simulink model "template"  (R2022b)
settings: Solver=VariableStepAuto  StartTime=0.0  StopTime=100  RelTol=1e-3
libraries: simulink_extras x3, aerolibanimutils x1, shared6dof x1
settings Model: Creator=alvar  LastModifiedBy=mluser

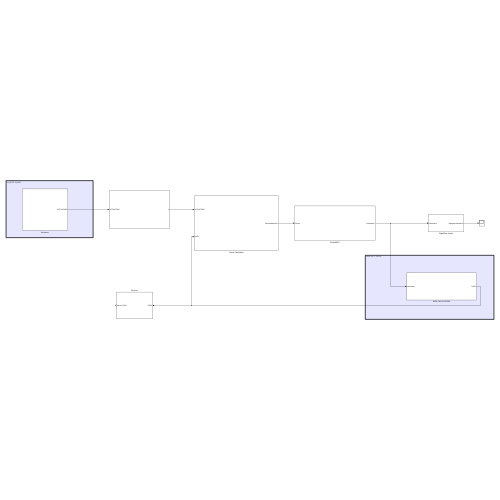
[thumbnail: Simulink's stored preview of the top-level diagram]
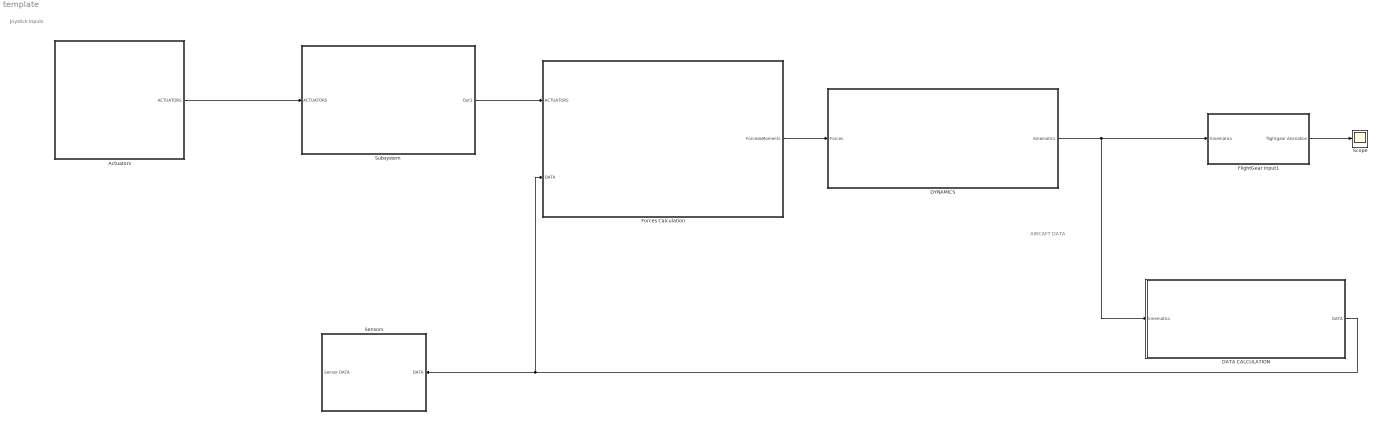
== system template ==
  note: Joystick Inputs
  note: AIRCAFT DATA
  Actuators : Subsystem
  DATA CALCULATION : Subsystem
  DYNAMICS : Subsystem
  FlightGear Input1 : Subsystem
  Forces Calculation : Subsystem
  Scope : Scope
  Sensors : Subsystem
  Subsystem : Subsystem
  wires:
  Forces Calculation/1(Forces&Moments) -> DYNAMICS/1(Forces)
  Actuators/1(ACTUATORS) -> Subsystem/1(ACTUATORS)
  DYNAMICS/1(Kinematics) -> FlightGear Input1/1(Kinematics), DATA CALCULATION/1(kinematics)
  DATA CALCULATION/1(DATA) -> Forces Calculation/2(DATA), Sensors/1(DATA)
  FlightGear Input1/1(flightgear Animation) -> Scope/1
  Subsystem/1(Out1) -> Forces Calculation/1(ACTUATORS)

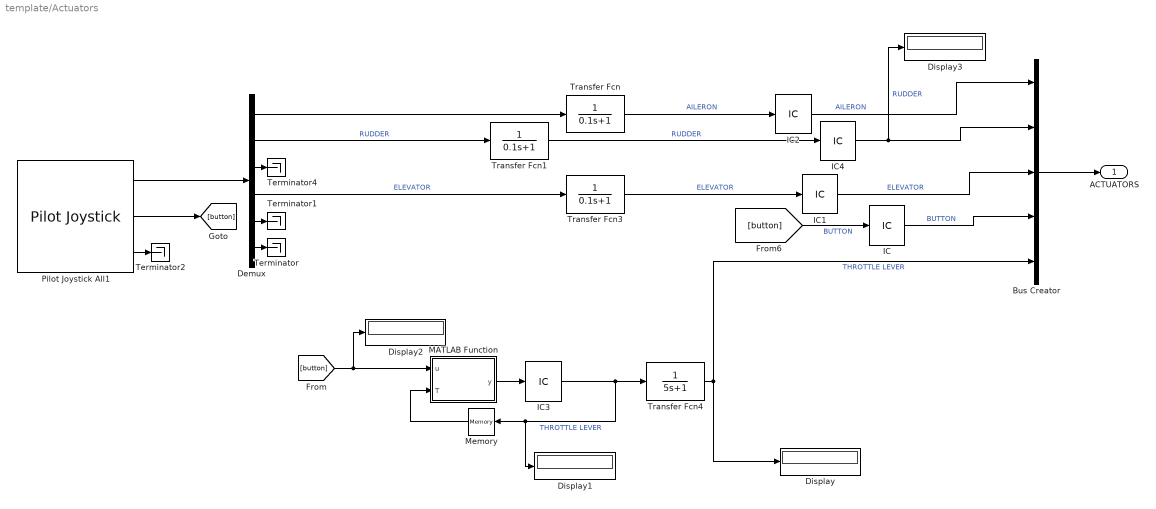
== system template/Actuators ==
  Bus Creator : BusCreator  Inputs=5
  Demux : Demux  Outputs=6
  Display{,1..3} (4 alike) : Display
  IC{,1..4} (5 alike) : InitialCondition  Value=0
  MATLAB Function : MATLAB Function  TreatAsAtomicUnit=on
  Memory : Memory
  Pilot Joystick All1 : aerolibanimutils/Pilot Joystick  JoystickID=Joystick1  OutputConfiguration=AllOutputs  SampleTime=1/30
      settings: LibrarySourceBlock=aerolibanimutils/Pilot Joystick All
  Terminator{,1..2,4} (4 alike) : Terminator
  Transfer Fcn : TransferFcn  Denominator=[0.1 1]
  Transfer Fcn1 : TransferFcn  Denominator=[0.1 1]
  Transfer Fcn3 : TransferFcn  Denominator=[0.1 1]
  Transfer Fcn4 : TransferFcn  Denominator=[5 1]
  ACTUATORS : Outport
  wires:
  Pilot Joystick All1/1 -> Demux/1
  Pilot Joystick All1/3 -> Terminator2/1
  Transfer Fcn3/1 -> IC1/1  "ELEVATOR"
  Pilot Joystick All1/2 -> [button]
  [button] -> IC/1  "BUTTON"
  Bus Creator/1 -> ACTUATORS/1
  IC/1 -> Bus Creator/4  "BUTTON"
  Transfer Fcn1/1 -> IC4/1  "RUDDER"
  Transfer Fcn/1 -> IC2/1  "AILERON"
  Demux/1 -> Transfer Fcn/1
  Demux/6 -> Terminator/1
  Demux/5 -> Terminator1/1
  Demux/4 -> Transfer Fcn3/1  "ELEVATOR"
  Demux/2 -> Transfer Fcn1/1  "RUDDER"
  Memory/1 -> MATLAB Function/2(T)
  IC3/1 -> Display1/1, Memory/1, Transfer Fcn4/1  "THROTTLE LEVER"
  MATLAB Function/1(y) -> IC3/1
  [button] -> Display2/1, MATLAB Function/1(u)
  Demux/3 -> Terminator4/1
  Transfer Fcn4/1 -> Display/1, Bus Creator/5  "THROTTLE LEVER"
  IC2/1 -> Bus Creator/1  "AILERON"
  IC4/1 -> Display3/1, Bus Creator/2  "RUDDER"
  IC1/1 -> Bus Creator/3  "ELEVATOR"

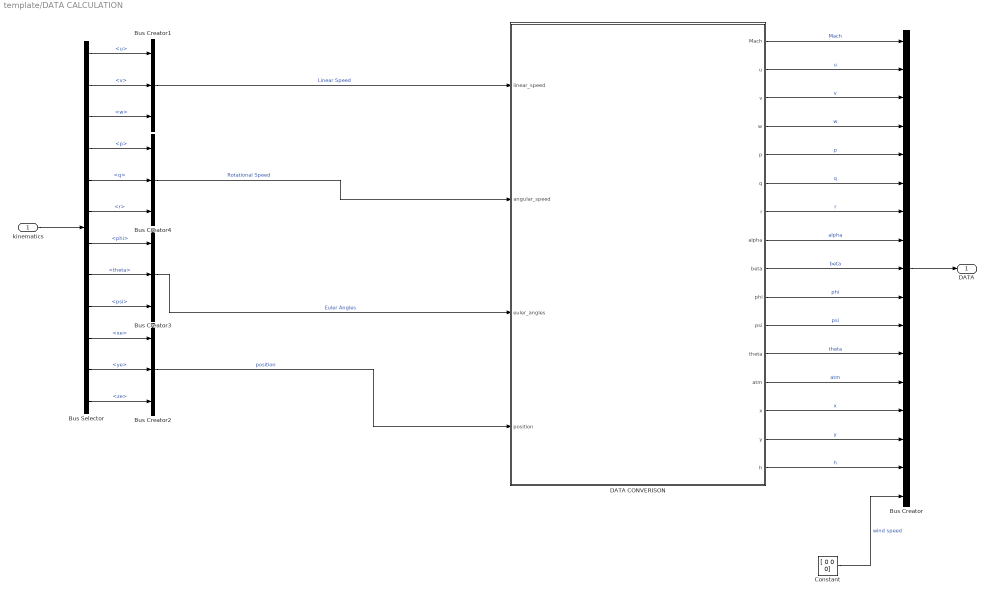
== system template/DATA CALCULATION ==
  kinematics : Inport
  Bus Creator : BusCreator  Inputs=17
  Bus Creator{1..4} (4 alike) : BusCreator  Inputs=3
  Bus Selector : BusSelector  OutputSignals=u,v,w,p,q,r,phi,theta,psi,xe,ye,ze
  Constant : Constant  Value=[ 0 0 0]
  DATA CONVERISON : MATLAB Function  TreatAsAtomicUnit=on
  DATA : Outport
  wires:
  kinematics/1 -> Bus Selector/1
  Bus Creator1/1 -> DATA CONVERISON/1(linear_speed)  "Linear Speed"
  Bus Creator4/1 -> DATA CONVERISON/2(angular_speed)  "Rotational Speed"
  Bus Creator3/1 -> DATA CONVERISON/3(euler_angles)  "Euler Angles"
  DATA CONVERISON/1(Mach) -> Bus Creator/1  "Mach"
  DATA CONVERISON/2(u) -> Bus Creator/2  "u"
  DATA CONVERISON/3(v) -> Bus Creator/3  "v"
  DATA CONVERISON/4(w) -> Bus Creator/4  "w"
  DATA CONVERISON/5(p) -> Bus Creator/5  "p"
  DATA CONVERISON/6(q) -> Bus Creator/6  "q"
  DATA CONVERISON/7(r) -> Bus Creator/7  "r"
  DATA CONVERISON/8(alpha) -> Bus Creator/8  "alpha"
  DATA CONVERISON/9(beta) -> Bus Creator/9  "beta"
  DATA CONVERISON/10(phi) -> Bus Creator/10  "phi"
  DATA CONVERISON/11(psi) -> Bus Creator/11  "psi"
  DATA CONVERISON/12(theta) -> Bus Creator/12  "theta"
  DATA CONVERISON/13(atm) -> Bus Creator/13  "atm"
  Bus Creator/1 -> DATA/1
  DATA CONVERISON/14(x) -> Bus Creator/14  "x"
  DATA CONVERISON/15(y) -> Bus Creator/15  "y"
  DATA CONVERISON/16(h) -> Bus Creator/16  "h"
  Bus Creator2/1 -> DATA CONVERISON/4(position)  "position"
  Bus Selector/1 -> Bus Creator1/1  "<u>"
  Bus Selector/2 -> Bus Creator1/2  "<v>"
  Bus Selector/3 -> Bus Creator1/3  "<w>"
  Bus Selector/10 -> Bus Creator2/1  "<xe>"
  Bus Selector/11 -> Bus Creator2/2  "<ye>"
  Bus Selector/12 -> Bus Creator2/3  "<ze>"
  Bus Selector/7 -> Bus Creator3/1  "<phi>"
  Bus Selector/8 -> Bus Creator3/2  "<theta>"
  Bus Selector/9 -> Bus Creator3/3  "<psi>"
  Bus Selector/4 -> Bus Creator4/1  "<p>"
  Bus Selector/5 -> Bus Creator4/2  "<q>"
  Bus Selector/6 -> Bus Creator4/3  "<r>"
  Constant/1 -> Bus Creator/17  "wind speed"

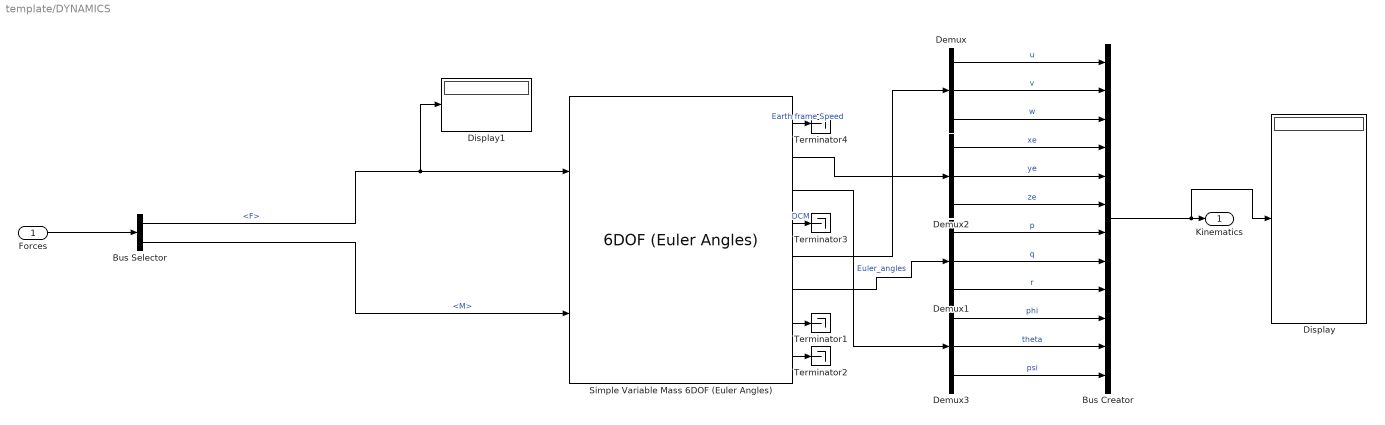
== system template/DYNAMICS ==
  Forces : Inport
  Bus Creator : BusCreator  Inputs=12
  Bus Selector : BusSelector  OutputSignals=F,M
  Demux{,1..3} (4 alike) : Demux  Outputs=3
  Display : Display
  Display1 : Display
  Simple Variable Mass 6DOF (Euler Angles) : shared6dof/6DOF (Euler Angles)  units=Metric (MKS)  mtype=Fixed  rep=Euler Angles  xme_0=[0 0 5000*0.3048]  Vm_0=[267.5, 0, 10]  eul_0=[0 0 0]  pm_0=[0 0 0]  mass_0=16284  mass_e=39500  mass_f=78000.0  inertia="[3.4573e+04 0 -1.3558e+03; 0  2.2588e+05 0;  -1.3558e+03 0 2.5354e+05]"  inertia_e=[1062400 3092400 4015300 0 104470 0]  inertia_f=[1062400 3092400 4015300 0 104470 0]  k_quat=1.0  vre_flag=off  abi_flag=off  aMode=0  xme_statename=''  Vm_statename=''  eul_statename=''  quat_statename=''  pm_statename=''  mass_statename=''
      settings: LibrarySourceBlock=aerolib6dof2/Simple Variable Mass 6DOF (Euler Angles)
  Terminator{1..4} (4 alike) : Terminator
  Kinematics : Outport
  wires:
  Simple Variable Mass 6DOF (Euler Angles)/6 -> Demux1/1
  Bus Selector/1 -> Display1/1, Simple Variable Mass 6DOF (Euler Angles)/1  "<F>"
  Bus Selector/2 -> Simple Variable Mass 6DOF (Euler Angles)/2  "<M>"
  Forces/1 -> Bus Selector/1
  Simple Variable Mass 6DOF (Euler Angles)/7 -> Terminator1/1
  Bus Creator/1 -> Display/1, Kinematics/1
  Simple Variable Mass 6DOF (Euler Angles)/8 -> Terminator2/1
  Demux/1 -> Bus Creator/1  "u"
  Demux/2 -> Bus Creator/2  "v"
  Demux/3 -> Bus Creator/3  "w"
  Demux1/1 -> Bus Creator/7  "p"
  Demux1/2 -> Bus Creator/8  "q"
  Demux1/3 -> Bus Creator/9  "r"
  Simple Variable Mass 6DOF (Euler Angles)/2 -> Demux2/1
  Demux2/1 -> Bus Creator/4  "xe"
  Demux2/2 -> Bus Creator/5  "ye"
  Demux2/3 -> Bus Creator/6  "ze"
  Simple Variable Mass 6DOF (Euler Angles)/5 -> Demux/1
  Demux3/1 -> Bus Creator/10  "phi"
  Demux3/2 -> Bus Creator/11  "theta"
  Demux3/3 -> Bus Creator/12  "psi"
  Simple Variable Mass 6DOF (Euler Angles)/4 -> Terminator3/1  "DCM"
  Simple Variable Mass 6DOF (Euler Angles)/1 -> Terminator4/1  "Earth frame Speed"
  Simple Variable Mass 6DOF (Euler Angles)/3 -> Demux3/1  "Euler_angles"

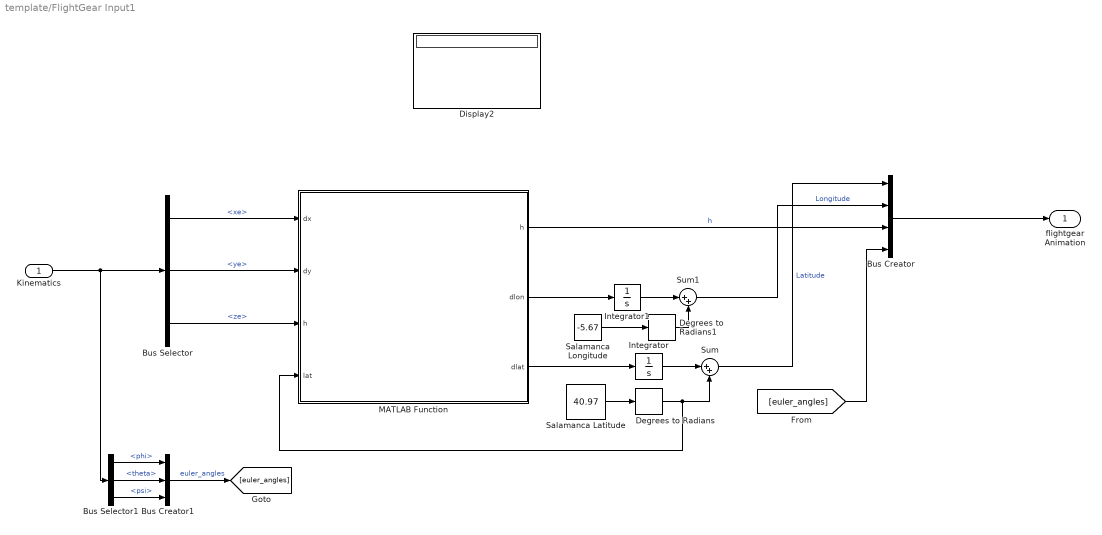
== system template/FlightGear Input1 ==
  Kinematics : Inport
  Bus Creator : BusCreator  Inputs=4
  Bus Creator1 : BusCreator  Inputs=3
  Bus Selector : BusSelector  OutputSignals=xe,ye,ze
  Bus Selector1 : BusSelector  OutputSignals=phi,theta,psi
  Degrees to Radians : simulink_extras/Transformations/Degrees to Radians
  Degrees to Radians1 : simulink_extras/Transformations/Degrees to Radians
  Display2 : Display
  Integrator : Integrator
  Integrator1 : Integrator
  MATLAB Function : MATLAB Function  TreatAsAtomicUnit=on
  Salamanca Latitude : Constant  Value=40.97
  Salamanca Longitude : Constant  Value=-5.67
  Sum : Sum  Inputs=|++
  Sum1 : Sum  Inputs=|++
  flightgear Animation : Outport
  wires:
  Bus Creator/1 -> flightgear Animation/1
  Integrator/1 -> Sum/1
  MATLAB Function/3(dlat) -> Integrator/1
  Salamanca Latitude/1 -> Degrees to Radians/1
  Degrees to Radians/1 -> MATLAB Function/4(lat), Sum/2
  Integrator1/1 -> Sum1/1
  MATLAB Function/2(dlon) -> Integrator1/1
  Salamanca Longitude/1 -> Degrees to Radians1/1
  Degrees to Radians1/1 -> Sum1/2
  Sum/1 -> Bus Creator/1  "Latitude"
  Sum1/1 -> Bus Creator/2  "Longitude"
  MATLAB Function/1(h) -> Bus Creator/3  "h"
  [euler_angles] -> Bus Creator/4
  Kinematics/1 -> Bus Selector1/1, Bus Selector/1
  Bus Selector/1 -> MATLAB Function/1(dx)  "<xe>"
  Bus Selector/2 -> MATLAB Function/2(dy)  "<ye>"
  Bus Selector/3 -> MATLAB Function/3("h ")  "<ze>"
  Bus Selector1/1 -> Bus Creator1/1  "<phi>"
  Bus Selector1/2 -> Bus Creator1/2  "<theta>"
  Bus Selector1/3 -> Bus Creator1/3  "<psi>"
  Bus Creator1/1 -> [euler_angles]  "euler_angles"

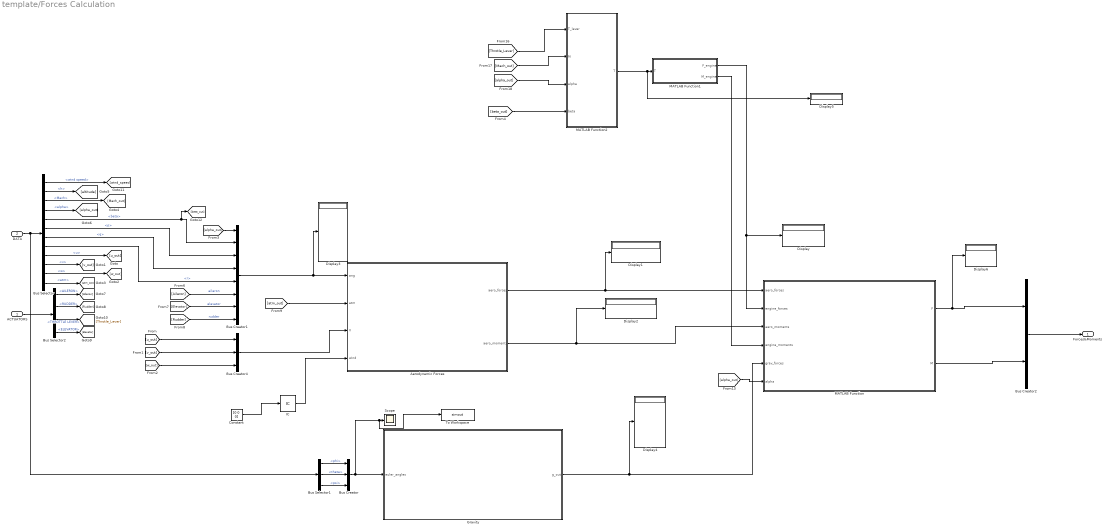
== system template/Forces Calculation ==
  ACTUATORS : Inport
  DATA : Inport  Port=2
  Aerodynamic Forces : MATLAB Function  TreatAsAtomicUnit=on
  Bus Creator : BusCreator  Inputs=3
  Bus Creator1 : BusCreator  Inputs=8
  Bus Creator2 : BusCreator  Inputs=2
  Bus Creator4 : BusCreator  Inputs=3
  Bus Selector : BusSelector  OutputSignals=wind speed,h,Mach,alpha,beta,p,q,r,u,v,w,atm
  Bus Selector1 : BusSelector  OutputSignals=phi,theta,psi
  Bus Selector2 : BusSelector  OutputSignals=AILERON,RUDDER,THROTTLE LEVER,ELEVATOR
  Constant : Constant  Value=[0 0 0]
  Display{,1..6} (7 alike) : Display
  Gravity : MATLAB Function  TreatAsAtomicUnit=on
  IC : InitialCondition  Value=[0 0 0]
  MATLAB Function : MATLAB Function  TreatAsAtomicUnit=on
  MATLAB Function1 : MATLAB Function  TreatAsAtomicUnit=on
  MATLAB Function2 : MATLAB Function  TreatAsAtomicUnit=on
  Scope : Scope
  To Workspace : ToWorkspace  VariableName=simout  SampleTime=-1
  Forces&Moments : Outport
  wires:
  [Rudder] -> Bus Creator1/8  "rudder"
  [alpha_out] -> MATLAB Function/6(alpha)
  Bus Selector/7 -> Bus Creator1/4  "<q>"
  Aerodynamic Forces/2(aero_moments) -> Display2/1, MATLAB Function/3(aero_moments)
  Bus Creator/1 -> To Workspace/1, Scope/1, Gravity/1(euler_angles)
  [atm_out] -> Aerodynamic Forces/2(atm)
  Aerodynamic Forces/1(aero_forces) -> Display1/1, MATLAB Function/1(aero_forces)
  MATLAB Function/2(M) -> Bus Creator2/2
  Bus Selector/8 -> Bus Creator1/5  "<r>"
  [alpha_out] -> MATLAB Function2/3(alpha)
  Bus Creator1/1 -> Display3/1, Aerodynamic Forces/1(ang)
  [Aileron] -> Bus Creator1/6  "aileron"
  MATLAB Function1/2(M_engine) -> MATLAB Function/4(engine_moments)
  [Mach_out] -> MATLAB Function2/2(M)
  Gravity/1(g_out) -> Display4/1, MATLAB Function/5(grav_forces)
  Bus Creator4/1 -> Aerodynamic Forces/3(V)
  Constant/1 -> IC/1
  MATLAB Function2/1(T) -> Display5/1, MATLAB Function1/1(T)
  MATLAB Function/1(F) -> Display6/1, Bus Creator2/1
  [Elevator] -> Bus Creator1/7  "elevator"
  DATA/1 -> Bus Selector1/1, Bus Selector/1
  Bus Selector/5 -> [beta_out], Bus Creator1/2  "<beta>"
  Bus Selector/6 -> Bus Creator1/3  "<p>"
  Bus Selector/9 -> [u_out]  "<u>"
  Bus Selector/10 -> [v_out]  "<v>"
  Bus Selector/11 -> [w_out]  "<w>"
  [u_out] -> Bus Creator4/1
  [v_out] -> Bus Creator4/2
  [w_out] -> Bus Creator4/3
  Bus Selector/12 -> [atm_out]  "<atm>"
  Bus Selector/3 -> [Mach_out]  "<Mach>"
  Bus Selector/2 -> [altitude]  "<h>"
  Bus Selector/4 -> [alpha_out]  "<alpha>"
  [alpha_out] -> Bus Creator1/1
  Bus Selector1/1 -> Bus Creator/1  "<phi>"
  Bus Selector1/3 -> Bus Creator/3  "<psi>"
  Bus Selector1/2 -> Bus Creator/2  "<theta>"
  ACTUATORS/1 -> Bus Selector2/1
  Bus Selector2/1 -> [Aileron]  "<AILERON>"
  Bus Selector2/2 -> [Rudder]  "<RUDDER>"
  Bus Selector2/3 -> [Throtle_Lever]  "<THROTTLE LEVER>"
  Bus Selector2/4 -> [Elevator]  "<ELEVATOR>"
  Bus Creator2/1 -> Forces&Moments/1
  Bus Selector/1 -> [wind_speed]  "<wind speed>"
  IC/1 -> Aerodynamic Forces/4(wind)
  MATLAB Function1/1(F_engine) -> MATLAB Function/2(engine_forces), Display/1
  [Throtle_Lever] -> MATLAB Function2/1(T_lever)
  [beta_out] -> MATLAB Function2/4(beta)

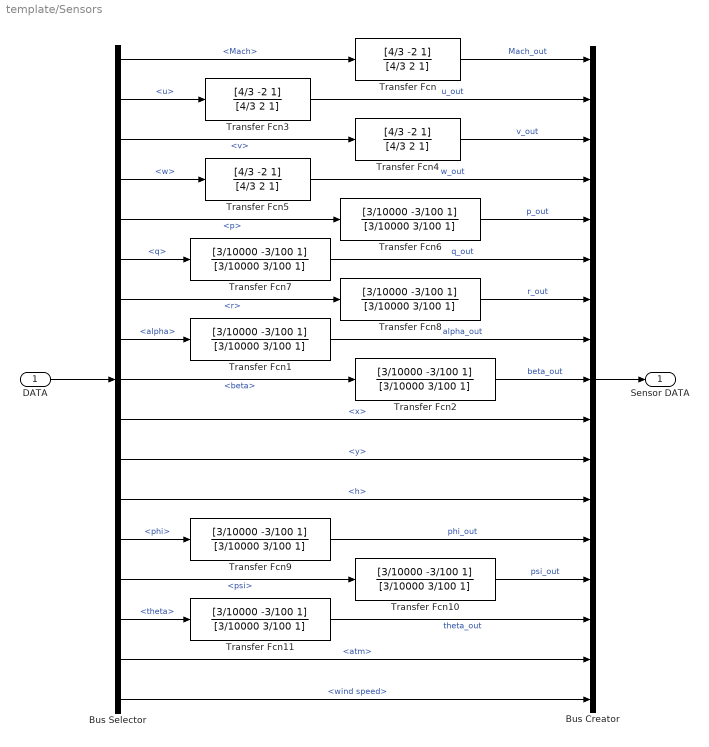
== system template/Sensors ==
  DATA : Inport
  Bus Creator : BusCreator  Inputs=17
  Bus Selector : BusSelector  OutputSignals=Mach,u,v,w,p,q,r,alpha,beta,x,y,h,phi,psi,theta,atm,wind speed
  Transfer Fcn{,3..5} (4 alike) : TransferFcn  Numerator=[4/3 -2 1]  Denominator=[4/3 2 1]
  Transfer Fcn{1..2,6..11} (8 alike) : TransferFcn  Numerator=[3/10000 -3/100 1]  Denominator=[3/10000 3/100 1]
  Sensor DATA : Outport
  wires:
  DATA/1 -> Bus Selector/1
  Bus Selector/14 -> Transfer Fcn10/1  "<psi>"
  Bus Selector/10 -> Bus Creator/10  "<x>"
  Transfer Fcn3/1 -> Bus Creator/2  "u_out"
  Transfer Fcn/1 -> Bus Creator/1  "Mach_out"
  Transfer Fcn6/1 -> Bus Creator/5  "p_out"
  Transfer Fcn4/1 -> Bus Creator/3  "v_out"
  Bus Selector/5 -> Transfer Fcn6/1  "<p>"
  Bus Selector/6 -> Transfer Fcn7/1  "<q>"
  Bus Selector/15 -> Transfer Fcn11/1  "<theta>"
  Bus Selector/13 -> Transfer Fcn9/1  "<phi>"
  Bus Selector/3 -> Transfer Fcn4/1  "<v>"
  Transfer Fcn11/1 -> Bus Creator/15  "theta_out"
  Transfer Fcn10/1 -> Bus Creator/14  "psi_out"
  Bus Selector/7 -> Transfer Fcn8/1  "<r>"
  Bus Selector/8 -> Transfer Fcn1/1  "<alpha>"
  Bus Selector/2 -> Transfer Fcn3/1  "<u>"
  Bus Selector/16 -> Bus Creator/16  "<atm>"
  Bus Selector/1 -> Transfer Fcn/1  "<Mach>"
  Bus Selector/9 -> Transfer Fcn2/1  "<beta>"
  Bus Selector/4 -> Transfer Fcn5/1  "<w>"
  Transfer Fcn1/1 -> Bus Creator/8  "alpha_out"
  Transfer Fcn5/1 -> Bus Creator/4  "w_out"
  Transfer Fcn7/1 -> Bus Creator/6  "q_out"
  Transfer Fcn8/1 -> Bus Creator/7  "r_out"
  Transfer Fcn9/1 -> Bus Creator/13  "phi_out"
  Transfer Fcn2/1 -> Bus Creator/9  "beta_out"
  Bus Creator/1 -> Sensor DATA/1
  Bus Selector/11 -> Bus Creator/11  "<y>"
  Bus Selector/12 -> Bus Creator/12  "<h>"
  Bus Selector/17 -> Bus Creator/17  "<wind speed>"

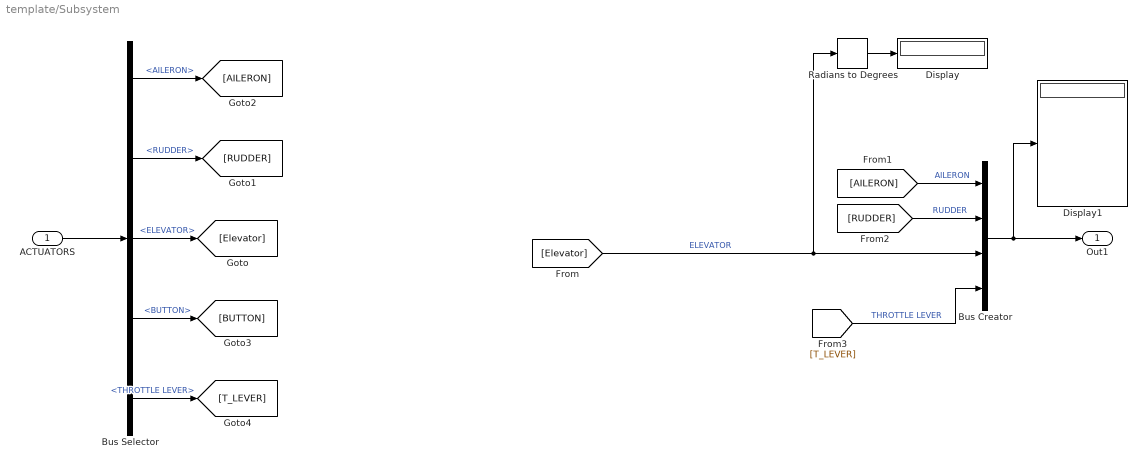
== system template/Subsystem ==
  ACTUATORS : Inport
  Bus Creator : BusCreator  Inputs=4
  Bus Selector : BusSelector  OutputSignals=AILERON,RUDDER,ELEVATOR,BUTTON,THROTTLE LEVER
  Display : Display
  Display1 : Display
  Radians to Degrees : simulink_extras/Transformations/Radians to Degrees
  Out1 : Outport
  wires:
  ACTUATORS/1 -> Bus Selector/1
  Bus Selector/1 -> [AILERON]  "<AILERON>"
  Bus Selector/2 -> [RUDDER]  "<RUDDER>"
  Bus Selector/3 -> [Elevator]  "<ELEVATOR>"
  Bus Selector/4 -> [BUTTON]  "<BUTTON>"
  [Elevator] -> Radians to Degrees/1, Bus Creator/3  "ELEVATOR"
  [RUDDER] -> Bus Creator/2  "RUDDER"
  [AILERON] -> Bus Creator/1  "AILERON"
  Bus Creator/1 -> Out1/1, Display1/1
  Bus Selector/5 -> [T_LEVER]  "<THROTTLE LEVER>"
  [T_LEVER] -> Bus Creator/4  "THROTTLE LEVER"
  Radians to Degrees/1 -> Display/1

== matlab function template/Forces Calculation/Gravity ==
  data: euler_angles input; g_out output
%% Gravity function
function g_out = gravity(euler_angles)
    mass = 78000; % kg % Decrease mass on each step
    phi = euler_angles(1);
    g=9.81;
    teta = euler_angles(2);
    g_out = zeros(1,6);
    g_out(1) = -g*sin(teta)*mass;
    g_out(2) = g*sin(phi)*cos(teta)*mass;
    g_out(3) = g*cos(phi)*cos(teta)*mass;
    g_out(4:6) = 0;

== matlab function template/FlightGear Input1/MATLAB Function ==
  data: h output; dlon output; dx input; dy input; h input; dlat output; lat input
function [h,dlon, dlat] = fcn(dx,dy,h,lat)
%% refining input
% dx = earth_frame_position(1);
% dy = earth_frame_position(2);
% h = earth_frame_position(3);

%% Model Parameters
a=6378137.0;
finv=298.257222101;
f=1/finv;
b=a*(1-f);
e2=1-(1-f)^2;
% https://es.mathworks.com/matlabcentral/fileexchange/15285-geodetic-toolbox
%% Model equations
v=a./sqrt(1-e2.*sin(lat).^2);
r=v.*(1-e2)./(1-e2.*sin(lat).^2);
dlat=dx./(r+h);
dlon=dy./cos(lat)./(v+h);

== matlab function template/Forces Calculation/Aerodynamic Forces ==
  data: ang input; aero_forces output; atm input; V input; aero_moments output; wind input
function [aero_forces, aero_moments] = aerodynamic_forces(ang,atm,V,wind)
%% Output Initialization
aero_forces = zeros(1, 3);
aero_forces_temp = zeros(1, 3);
aero_moments = zeros(1, 3);
%% Data definition
V = V + wind;
S_wb = 608*0.3048^2; % Wing surface
b = 42.8*0.3048; % wingspan
CMA = 15.94*0.3048; % Aerodynamic mean chord
% ang(6:7) = 0;
c_0 = [0.0077 0 0.327 0 0 0 0]; % Non perturbance coefficients [cd0, cy0, cL0, cl0, cm0, cn0]
c_alpha = [1.0429 0 5.9078 0 -10.8294 0 0]; % alpha derivative coefficients [cd_alpha, cy_alpha, cL_alpha, cl_alpha, cm_alpha, cn_alpha]
c_beta = [0 -0.5514 0 -0.0493 0 0.10047]; % beta derivative coefficients [cd_beta, cy_beta, cL_beta, cl_beta, cm_beta, cn_beta]
c_p = [0 0 0 -0.41956 0 -0.017505]; % p derivative coefficients [cd_p, cy_p, cL_p, cl_p, cm_p, cn_p]
c_q = [0 0 33.7202 0 -111.4021 0]; % q derivative coefficients [cd_q, cy_q, cL_q, cl_q, cm_q, cn_q]
c_r = [0 0.28399 0 0.09915 0 -0.22535]; % r derivative coefficients [cd_r, cy_r, cL_r, cl_r, cm_r, cn_r]
c_aileron = [0 0 0 0.159 0 -0.00637]; % delta derivative coefficients [cd_delta, cy_delta, cL_delta, cl_delta, cm_delta, cn_delta]
c_rudder = [0 0.115021 0 0.007089 0 -0.6431]; % delta derivative coefficients [cd_delta, cy_delta, cL_delta, cl_delta, cm_delta, cn_delta]
c_elevator = [0 0 -0.2784e-4 0 -3.933 0]; % delta derivative coefficients [cd_delta, cy_delta, cL_delta, cl_delta, cm_delta, cn_delta]

%% Data preparation
% first calculations
us = norm(V);
% Dynamic Pressure
q = 0.5 * atm(3) * us^2;
ang(3) = ang(3) * b / (2 * us);
ang(4) = ang(4) * CMA / (2 * us);
ang(5) = ang(5) * b / (2 * us);
alpha=ang(1);beta=ang(2); p_=ang(3);q_=ang(4);r_=ang(5);aileron=ang(6);
elevator=ang(7);rudder=ang(8);
%% Aerodynamic forces Computation
aero_forces_temp(1) = q * S_wb * (0.05 + 0.210 * alpha);
aero_forces_temp(2) = q * S_wb * (-0.87 * beta + 0.06*p_ + 0.38*r_ - 0.006*aileron);
aero_forces_temp(3) = q * S_wb * (0.075 + 4.17*alpha + 0.36*elevator);

aero_forces(1) = -aero_forces_temp(1) * cos(alpha) + aero_forces_temp(3) * sin(alpha);
aero_forces(2) = aero_forces_temp(2);
aero_forces(3) = -aero_forces_temp(3)*cos(alpha) - aero_forces_temp(1)*sin(alpha);
%% Aerodynamic Moments Computation
aero_moments(1) = q * S_wb* b * (-0.057*beta - 0.19*p_ + 0.03*r_ + 0.027*aileron - 0.004*rudder);
aero_moments(2) = q * S_wb * CMA * (-0.37*alpha -3.96*q_ - 0.45*elevator);
aero_moments(3) = q * S_wb * b * (0.14*beta - 0.02*p_ - 0.28*r_ + 0.0097*aileron + 0.094*rudder);

== matlab function template/Forces Calculation/MATLAB Function ==
  data: aero_forces input; engine_forces input; F output; aero_moments input; engine_moments input; grav_forces input; alpha input; M output
function [F,M] = forces_wrapper(aero_forces,engine_forces,aero_moments,engine_moments,grav_forces,alpha)
F=zeros(3,1);
M=zeros(3,1);
% F(1) = (aero_forces(3) * sin(alpha) - aero_forces(1) * cos(alpha) + grav_forces(1) + engine_forces(1)); % Add lg
% F(2) = (aero_forces(2) + grav_forces(2) + engine_forces(2)); % Add lg
% F(3) = (-aero_forces(3) * cos(alpha) - aero_forces(1) * sin(alpha) + grav_forces(3) + engine_forces(3)); % Add lg
F(1)=aero_forces(1)+grav_forces(1)+engine_forces(1);
F(2)=aero_forces(2)+grav_forces(2)+engine_forces(2);
F(3)=aero_forces(3)+grav_forces(3)+engine_forces(3);
M(1) = (aero_moments(1) + engine_moments(1) + grav_forces(4)); % Add lg
M(2) = (aero_moments(2) + engine_moments(2) + grav_forces(5)); % Add lg
M(3) = (aero_moments(3) + engine_moments(3) + grav_forces(6)); % Add lg

== matlab function template/Forces Calculation/MATLAB Function1 ==
  data: T input; F_engine output; M_engine output
function [F_engine, M_engine] = Engine_model(T)
F_engine = [2*T 0 0];
M_engine = [0 0 0];

== matlab function template/Forces Calculation/MATLAB Function2 ==
  data: T_lever input; T output; M input; alpha input; beta input
function T = engine(T_lever,M,alpha,beta)
T_max = 60000;
T = 2*M*cos(alpha)*cos(beta)*T_max*T_lever^4;

== matlab function template/Actuators/MATLAB Function ==
  data: u input; y output; T input
function y = fcn(u,T)
if u == 8
    y = T + 0.000000005;
elseif u==2
    y = T - 0.000000005;
else
    y=T;
end    
% if y>1 
%     y = 1;
% elseif y<0
%     y = 0;
% end

== matlab function template/DATA CALCULATION/DATA CONVERISON ==
  data: linear_speed input; Mach output; angular_speed input; euler_angles input; u output; v output; w output; p output; q output; r output; alpha output; beta output; phi output; psi output; theta output; atm output; x output; position input; y output; h output
function [Mach,u,v,w,p,q,r,alpha,beta,phi,psi,theta,atm,x,y,h] = sim_in_out(linear_speed,angular_speed,euler_angles,position)

    u = linear_speed(1);
    v = linear_speed(2);
    w = linear_speed(3);
    V = norm([u,v,w]);
    p = angular_speed(1);
    q = angular_speed(2);
    r = angular_speed(3);
    phi = euler_angles(1);
    psi = euler_angles(3);
    theta = euler_angles(2);
    atm = atmospheric_model(position(3));
    x=position(1);
    y=position(2);
    h=position(3);
    alpha = atan2(w,u);
    beta = atan(v/V);
    Mach = V/atm(4);
